simulink model "main_sys_v2_1"  (R2015a)
settings: Solver=ode23  StartTime=0.0  StopTime=Tfin  RelTol=1e-5  AbsTol=1e-5
undefined symbols (not defined in the file): init, K, param, x, x_dot, y, y_dot
settings Model: Creator=jesus  LastModifiedBy=jesus
settings SolverCC: InitialStep=1e-7  SolverResetMethod=Robust
settings DataIOCC: SaveState=on

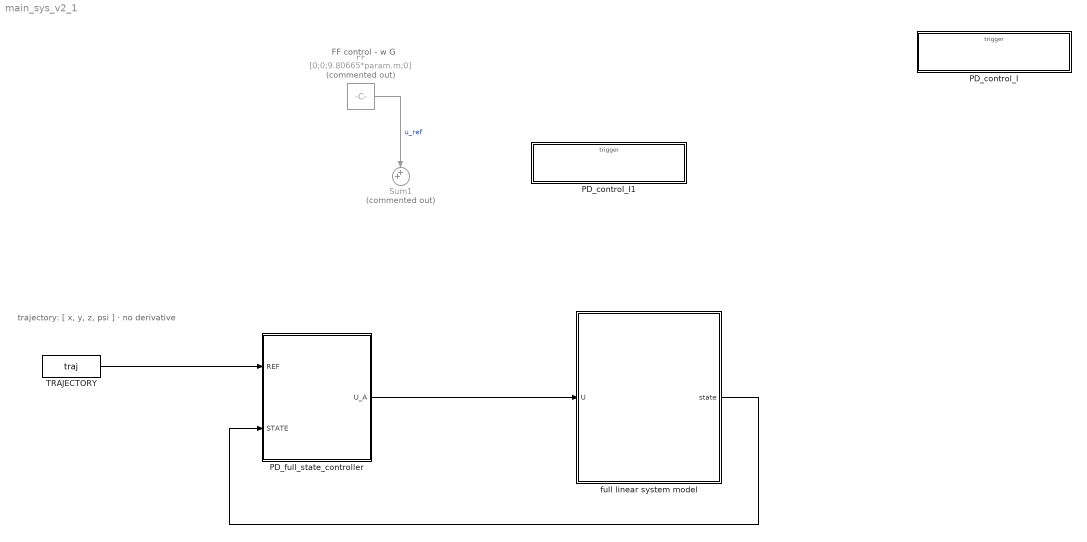
== system main_sys_v2_1 ==
  note: trajectory: [ x, y, z, psi ]
      |  · no derivative
  note: FF control - w G
  FF : Constant  Commented=on  Value=[0;0;9.80665*param.m;0]
  PD_control_I : Subsystem  TreatAsAtomicUnit=on
  PD_control_I1 : Subsystem  TreatAsAtomicUnit=on
  PD_full_state_controller : Subsystem
  Sum1 : Sum  Commented=on  Inputs=++|
  TRAJECTORY : FromWorkspace  VariableName=traj  SampleTime=param.hs  Interpolate=off  OutputAfterFinalValue=Setting to zero
  full linear system model : Subsystem
  wires:
  FF/1 -> Sum1/1  "u_ref"
  TRAJECTORY/1 -> PD_full_state_controller/1(REF)
  full linear system model/1(state) -> PD_full_state_controller/2(STATE)
  PD_full_state_controller/1(U_A) -> full linear system model/1(U)

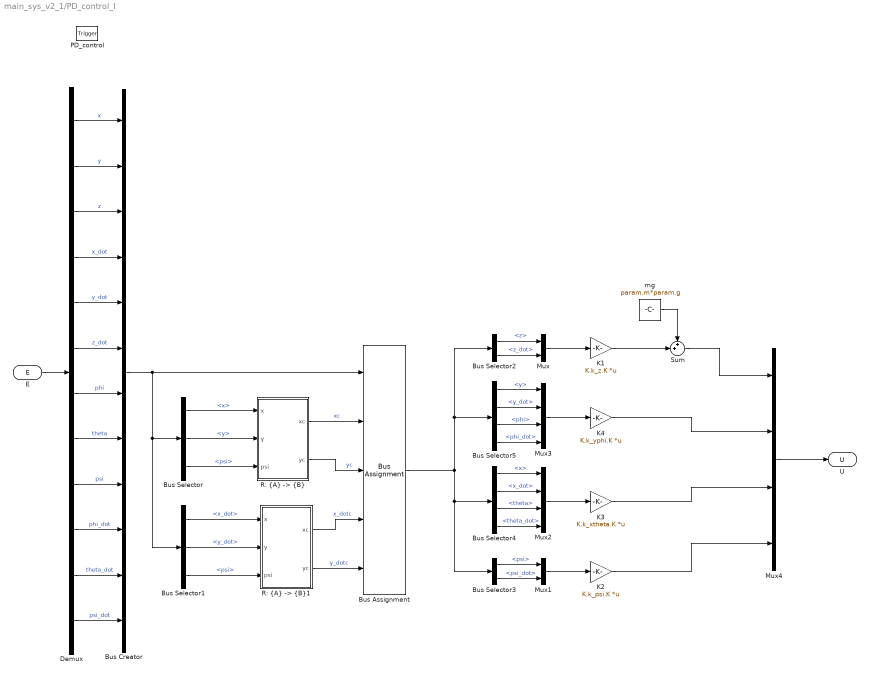
== system main_sys_v2_1/PD_control_I ==
  PD_control : TriggerPort  TriggerType=function-call  IsSimulinkFunction=on  FunctionName=PD_control
  Bus Assignment : BusAssignment  AssignedSignals=x,y,x_dot,y_dot
  Bus Creator : BusCreator  Inputs=12
  Bus Selector : BusSelector  OutputSignals=x,y,psi
  Bus Selector1 : BusSelector  OutputSignals=x_dot,y_dot,psi
  Bus Selector2 : BusSelector  OutputSignals=z,z_dot
  Bus Selector3 : BusSelector  OutputSignals=psi,psi_dot
  Bus Selector4 : BusSelector  OutputSignals=x,x_dot,theta,theta_dot
  Bus Selector5 : BusSelector  OutputSignals=y,y_dot,phi,phi_dot
  Demux : Demux  Outputs=12
  K1 : Gain  Gain=K.k_z.K  Multiplication=Matrix(K*u)
  K2 : Gain  Gain=K.k_psi.K  Multiplication=Matrix(K*u)
  K3 : Gain  Gain=K.k_xtheta.K  Multiplication=Matrix(K*u)
  K4 : Gain  Gain=K.k_yphi.K  Multiplication=Matrix(K*u)
  Mux : Mux  Inputs=2
  Mux1 : Mux  Inputs=2
  Mux2 : Mux
  Mux3 : Mux
  Mux4 : Mux
  "R: {A} -> {B}" : MATLAB Function  TreatAsAtomicUnit=on
  "R: {A} -> {B}1" : MATLAB Function  TreatAsAtomicUnit=on
  Sum : Sum  Inputs=++|
  mg : Constant  Value=param.m*param.g  SampleTime=-1
  E : ArgIn  DisableCoverage=on  PortDimensions=12  ArgumentName=E
  U : ArgOut  DisableCoverage=on  PortDimensions=4  ArgumentName=U
  wires:
  E/1 -> Demux/1
  Demux/1 -> Bus Creator/1  "x"
  Demux/2 -> Bus Creator/2  "y"
  Demux/12 -> Bus Creator/12  "psi_dot"
  Demux/7 -> Bus Creator/7  "phi"
  Demux/8 -> Bus Creator/8  "theta"
  Demux/3 -> Bus Creator/3  "z"
  Demux/4 -> Bus Creator/4  "x_dot"
  Demux/5 -> Bus Creator/5  "y_dot"
  Demux/6 -> Bus Creator/6  "z_dot"
  Demux/9 -> Bus Creator/9  "psi"
  Demux/10 -> Bus Creator/10  "phi_dot"
  Demux/11 -> Bus Creator/11  "theta_dot"
  Bus Selector/1 -> "R: {A} -> {B}"/1(x)  "<x>"
  Bus Selector/2 -> "R: {A} -> {B}"/2(y)  "<y>"
  Bus Selector/3 -> "R: {A} -> {B}"/3(psi)  "<psi>"
  "R: {A} -> {B}"/1(xc) -> Bus Assignment/2  "xc"
  "R: {A} -> {B}"/2(yc) -> Bus Assignment/3  "yc"
  Bus Creator/1 -> Bus Assignment/1, Bus Selector/1, Bus Selector1/1
  Bus Selector1/1 -> "R: {A} -> {B}1"/1(x)  "<x_dot>"
  Bus Selector1/2 -> "R: {A} -> {B}1"/2(y)  "<y_dot>"
  Bus Selector1/3 -> "R: {A} -> {B}1"/3(psi)  "<psi>"
  "R: {A} -> {B}1"/1(xc) -> Bus Assignment/4  "x_dotc"
  "R: {A} -> {B}1"/2(yc) -> Bus Assignment/5  "y_dotc"
  Bus Assignment/1 -> Bus Selector5/1, Bus Selector2/1, Bus Selector3/1, Bus Selector4/1
  Bus Selector2/1 -> Mux/1  "<z>"
  Bus Selector2/2 -> Mux/2  "<z_dot>"
  Bus Selector3/1 -> Mux1/1  "<psi>"
  Bus Selector3/2 -> Mux1/2  "<psi_dot>"
  Bus Selector5/1 -> Mux3/1  "<y>"
  Bus Selector5/2 -> Mux3/2  "<y_dot>"
  Bus Selector5/3 -> Mux3/3  "<phi>"
  Bus Selector5/4 -> Mux3/4  "<phi_dot>"
  Bus Selector4/4 -> Mux2/4  "<theta_dot>"
  Bus Selector4/3 -> Mux2/3  "<theta>"
  Bus Selector4/2 -> Mux2/2  "<x_dot>"
  Bus Selector4/1 -> Mux2/1  "<x>"
  Mux2/1 -> K3/1
  Mux1/1 -> K2/1
  Mux/1 -> K1/1
  Mux3/1 -> K4/1
  Mux4/1 -> U/1
  Sum/1 -> Mux4/1
  K1/1 -> Sum/2
  mg/1 -> Sum/1
  K4/1 -> Mux4/2
  K3/1 -> Mux4/3
  K2/1 -> Mux4/4

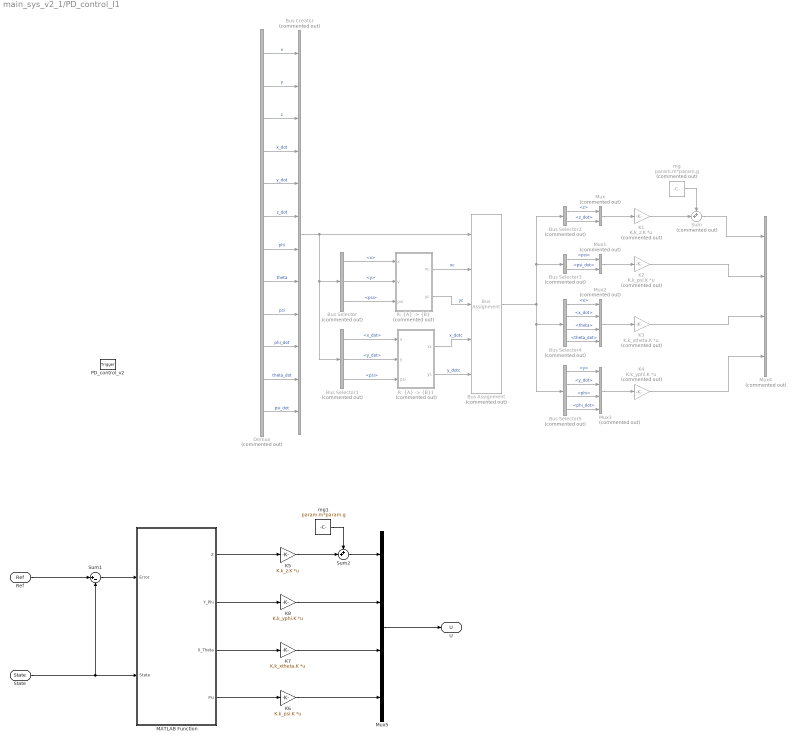
== system main_sys_v2_1/PD_control_I1 ==
  PD_control_v2 : TriggerPort  TriggerType=function-call  IsSimulinkFunction=on  FunctionName=PD_control_v2
  Bus Assignment : BusAssignment  Commented=on  AssignedSignals=x,y,x_dot,y_dot
  Bus Creator : BusCreator  Commented=on  Inputs=12
  Bus Selector : BusSelector  Commented=on  OutputSignals=x,y,psi
  Bus Selector1 : BusSelector  Commented=on  OutputSignals=x_dot,y_dot,psi
  Bus Selector2 : BusSelector  Commented=on  OutputSignals=z,z_dot
  Bus Selector3 : BusSelector  Commented=on  OutputSignals=psi,psi_dot
  Bus Selector4 : BusSelector  Commented=on  OutputSignals=x,x_dot,theta,theta_dot
  Bus Selector5 : BusSelector  Commented=on  OutputSignals=y,y_dot,phi,phi_dot
  Demux : Demux  Commented=on  Outputs=12
  K1 : Gain  Commented=on  Gain=K.k_z.K  Multiplication=Matrix(K*u)
  K2 : Gain  Commented=on  Gain=K.k_psi.K  Multiplication=Matrix(K*u)
  K3 : Gain  Commented=on  Gain=K.k_xtheta.K  Multiplication=Matrix(K*u)
  K4 : Gain  Commented=on  Gain=K.k_yphi.K  Multiplication=Matrix(K*u)
  K5 : Gain  Gain=K.k_z.K  Multiplication=Matrix(K*u)
  K6 : Gain  Gain=K.k_psi.K  Multiplication=Matrix(K*u)
  K7 : Gain  Gain=K.k_xtheta.K  Multiplication=Matrix(K*u)
  K8 : Gain  Gain=K.k_yphi.K  Multiplication=Matrix(K*u)
  MATLAB Function : MATLAB Function  TreatAsAtomicUnit=on
  Mux : Mux  Commented=on  Inputs=2
  Mux1 : Mux  Commented=on  Inputs=2
  Mux2 : Mux  Commented=on
  Mux3 : Mux  Commented=on
  Mux4 : Mux  Commented=on
  Mux5 : Mux
  "R: {A} -> {B}" : MATLAB Function  Commented=on  TreatAsAtomicUnit=on
  "R: {A} -> {B}1" : MATLAB Function  Commented=on  TreatAsAtomicUnit=on
  Sum : Sum  Commented=on  Inputs=++|
  Sum1 : Sum  Inputs=|+-
  Sum2 : Sum  Inputs=++|
  mg : Constant  Commented=on  Value=param.m*param.g  SampleTime=-1
  mg1 : Constant  Value=param.m*param.g  SampleTime=-1
  Ref : ArgIn  DisableCoverage=on  PortDimensions=12  ArgumentName=Ref
  State : ArgIn  DisableCoverage=on  Port=2  PortDimensions=12  ArgumentName=State
  U : ArgOut  DisableCoverage=on  PortDimensions=4  ArgumentName=U
  wires:
  Demux/1 -> Bus Creator/1  "x"
  Demux/2 -> Bus Creator/2  "y"
  Demux/12 -> Bus Creator/12  "psi_dot"
  Demux/7 -> Bus Creator/7  "phi"
  Demux/8 -> Bus Creator/8  "theta"
  Demux/3 -> Bus Creator/3  "z"
  Demux/4 -> Bus Creator/4  "x_dot"
  Demux/5 -> Bus Creator/5  "y_dot"
  Demux/6 -> Bus Creator/6  "z_dot"
  Demux/9 -> Bus Creator/9  "psi"
  Demux/10 -> Bus Creator/10  "phi_dot"
  Demux/11 -> Bus Creator/11  "theta_dot"
  Bus Selector/1 -> "R: {A} -> {B}"/1(x)  "<x>"
  Bus Selector/2 -> "R: {A} -> {B}"/2(y)  "<y>"
  Bus Selector/3 -> "R: {A} -> {B}"/3(psi)  "<psi>"
  "R: {A} -> {B}"/1(xc) -> Bus Assignment/2  "xc"
  "R: {A} -> {B}"/2(yc) -> Bus Assignment/3  "yc"
  Bus Creator/1 -> Bus Assignment/1, Bus Selector/1, Bus Selector1/1
  Bus Selector1/1 -> "R: {A} -> {B}1"/1(x)  "<x_dot>"
  Bus Selector1/2 -> "R: {A} -> {B}1"/2(y)  "<y_dot>"
  Bus Selector1/3 -> "R: {A} -> {B}1"/3(psi)  "<psi>"
  "R: {A} -> {B}1"/1(xc) -> Bus Assignment/4  "x_dotc"
  "R: {A} -> {B}1"/2(yc) -> Bus Assignment/5  "y_dotc"
  Bus Assignment/1 -> Bus Selector2/1, Bus Selector3/1, Bus Selector5/1, Bus Selector4/1
  Bus Selector2/1 -> Mux/1  "<z>"
  Bus Selector2/2 -> Mux/2  "<z_dot>"
  Bus Selector3/1 -> Mux1/1  "<psi>"
  Bus Selector3/2 -> Mux1/2  "<psi_dot>"
  Bus Selector5/1 -> Mux3/1  "<y>"
  Bus Selector5/2 -> Mux3/2  "<y_dot>"
  Bus Selector5/3 -> Mux3/3  "<phi>"
  Bus Selector5/4 -> Mux3/4  "<phi_dot>"
  Bus Selector4/4 -> Mux2/4  "<theta_dot>"
  Bus Selector4/3 -> Mux2/3  "<theta>"
  Bus Selector4/2 -> Mux2/2  "<x_dot>"
  Bus Selector4/1 -> Mux2/1  "<x>"
  Mux2/1 -> K3/1
  Mux1/1 -> K2/1
  Mux/1 -> K1/1
  Mux3/1 -> K4/1
  K3/1 -> Mux4/3
  K2/1 -> Mux4/2
  K4/1 -> Mux4/4
  Sum/1 -> Mux4/1
  K1/1 -> Sum/2
  mg/1 -> Sum/1
  Ref/1 -> Sum1/1
  State/1 -> Sum1/2, MATLAB Function/2(State)
  Sum1/1 -> MATLAB Function/1(Error)
  MATLAB Function/4(Psi) -> K6/1
  MATLAB Function/1(Z) -> K5/1
  MATLAB Function/3(X_Theta) -> K7/1
  MATLAB Function/2(Y_Phi) -> K8/1
  K5/1 -> Sum2/2
  mg1/1 -> Sum2/1
  K8/1 -> Mux5/2
  K7/1 -> Mux5/3
  K6/1 -> Mux5/4
  Sum2/1 -> Mux5/1
  Mux5/1 -> U/1

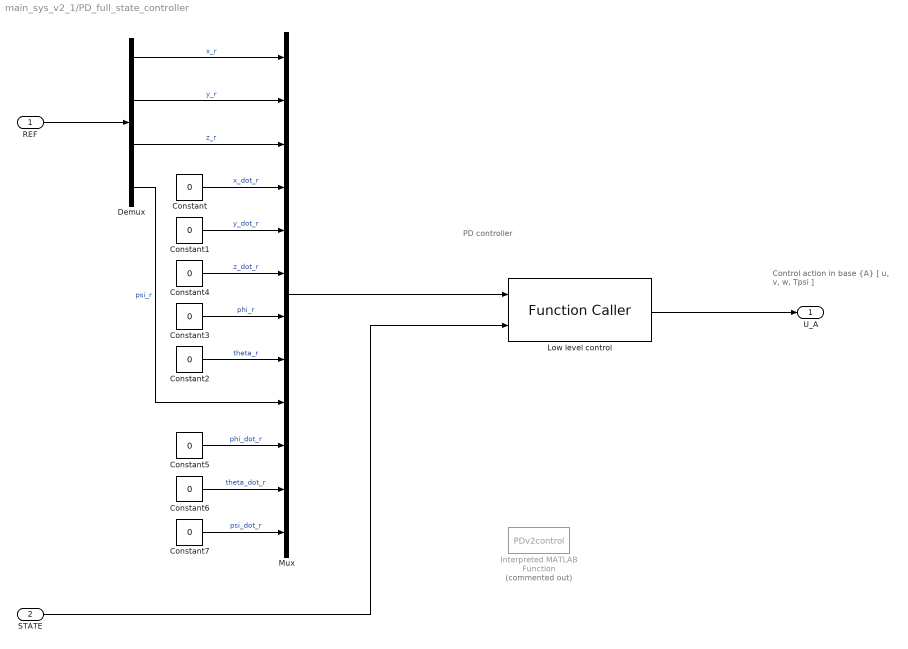
== system main_sys_v2_1/PD_full_state_controller ==
  note: Control action
      |    in base {A}
      |
      |
      |
      |
      | [ u, v, w, Tpsi ]
  note: PD controller
  REF : Inport
  STATE : Inport  Port=2
  Constant{,1..7} (8 alike) : Constant  Value=0
  Demux : Demux
  Interpreted MATLAB Function : MATLABFcn  Commented=on  MATLABFcn=PDv2control  OutputDimensions=4
  Low level control : FunctionCaller  FunctionPrototype=U = PD_control_v2(Ref,State)
  Mux : Mux  Inputs=12
  U_A : Outport
  wires:
  REF/1 -> Demux/1
  Demux/1 -> Mux/1  "x_r"
  Demux/2 -> Mux/2  "y_r"
  Demux/3 -> Mux/3  "z_r"
  STATE/1 -> Low level control/2
  Constant5/1 -> Mux/10  "phi_dot_r"
  Constant6/1 -> Mux/11  "theta_dot_r"
  Constant7/1 -> Mux/12  "psi_dot_r"
  Mux/1 -> Low level control/1
  Low level control/1 -> U_A/1
  Constant4/1 -> Mux/6  "z_dot_r"
  Constant1/1 -> Mux/5  "y_dot_r"
  Constant/1 -> Mux/4  "x_dot_r"
  Demux/4 -> Mux/9  "psi_r"
  Constant2/1 -> Mux/8  "theta_r"
  Constant3/1 -> Mux/7  "phi_r"

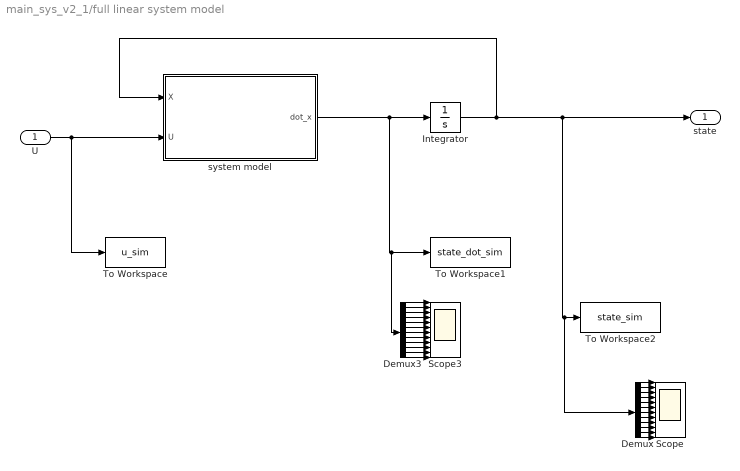
== system main_sys_v2_1/full linear system model ==
  U : Inport
  Demux : Demux  Outputs=12
  Demux3 : Demux  Outputs=12
  Integrator : Integrator  InitialCondition=init.full
  Scope : Scope  NumInputPorts=12
      settings: YMin=-5~-5~-5~-5~-5~-5~-5~-5~-5~-5~-5~-5  YMax=5~5~5~5~5~5~5~5~5~5~5~5
  Scope3 : Scope  NumInputPorts=12
      settings: YMin=-5~-5~-5~-5~-5~-5~-5~-5~-5~-5~-5~-5  YMax=5~5~5~5~5~5~5~5~5~5~5~5  SaveName=ScopeData3
  To Workspace : ToWorkspace  VariableName=u_sim  SaveFormat=Structure With Time  SampleTime=-1
  To Workspace1 : ToWorkspace  VariableName=state_dot_sim  SaveFormat=Structure With Time  SampleTime=-1
  To Workspace2 : ToWorkspace  VariableName=state_sim  SaveFormat=Structure With Time  SampleTime=-1
  system model : MATLAB Function  TreatAsAtomicUnit=on
  state : Outport
  wires:
  U/1 -> system model/2(U), To Workspace/1
  Integrator/1 -> state/1, Demux/1, To Workspace2/1, system model/1(X)
  system model/1(dot_x) -> Integrator/1, Demux3/1, To Workspace1/1
  Demux/1 -> Scope/1
  Demux/2 -> Scope/2
  Demux/3 -> Scope/3
  Demux/4 -> Scope/4
  Demux/5 -> Scope/5
  Demux/6 -> Scope/6
  Demux/7 -> Scope/7
  Demux/8 -> Scope/8
  Demux/9 -> Scope/9
  Demux/10 -> Scope/10
  Demux/11 -> Scope/11
  Demux/12 -> Scope/12
  Demux3/1 -> Scope3/1
  Demux3/2 -> Scope3/2
  Demux3/3 -> Scope3/3
  Demux3/4 -> Scope3/4
  Demux3/5 -> Scope3/5
  Demux3/6 -> Scope3/6
  Demux3/7 -> Scope3/7
  Demux3/8 -> Scope3/8
  Demux3/9 -> Scope3/9
  Demux3/10 -> Scope3/10
  Demux3/11 -> Scope3/11
  Demux3/12 -> Scope3/12

== matlab function main_sys_v2_1/PD_control_I/R: {A} -> {B} ==
  data: x input; y input; psi input; xc output; yc output
function [xc, yc] = fcn(x, y, psi)
%#codegen
% Change in cordenates from fixed frame {A} to body frame {B} of position
%  state coordenates
% · apply rotation matrix over phi (vertical) to [x] and [y]
% · the references are given in fix frame {A}, input [u] is computed in
%   body frame {B}

R = [ cos(psi) sin(psi)
     -sin(psi) cos(psi)];
a = R * [x, y]';
xc = a(1);
yc = a(2);

== matlab function main_sys_v2_1/full linear system model/system model ==
  data: X input; U input; dot_x output
function dot_x = eq_quad_lin( X, U )
% Computes the linearized dynamics model of a quadcopter

% State
    x      = X(1);     Vx   = X(4);
    y      = X(2);     Vy   = X(5);
    z      = X(3);     Vz   = X(6);

    phi    = X(7);     p    = X(10);
    theta  = X(8);     q    = X(11);
    psi    = X(9);     r    = X(12);

% Inputs
    T  = U(1);       Tphi   = U(2);
                     Ttheta = U(3);
                     Tpsi   = U(4);
                
% parameters
     m = 0.429;    g = 9.80665;   
     Ix = 0.0022375681;  Iy = 0.002985236;  Iz = 0.00480374;
    
% Equations
dot_x = zeros(12,1);

dot_x(1)  = Vx;
dot_x(2)  = Vy;
dot_x(3)  = Vz;

dot_x(4)  = -(T/m) * ( theta );
dot_x(5)  = +(T/m) * ( phi );
dot_x(6)  = -(T/m) + g;

dot_x(7)  = p;
dot_x(8)  = q;
dot_x(9)  = r;

dot_x(10) = Tphi   / Ix;
dot_x(11) = Ttheta / Iy;
dot_x(12) = Tpsi   / Iz;

end

== matlab function main_sys_v2_1/PD_control_I/R: {A} -> {B}1 ==
  data: x input; y input; psi input; xc output; yc output
function [xc, yc] = fcn(x, y, psi)
%#codegen
% Change in cordenates from fixed frame {A} to body frame {B} of position
%  state coordenates
% · apply rotation matrix over phi (vertical) to [x] and [y]
% · the references are given in fix frame {A}, input [u] is computed in
%   body frame {B}

R = [ cos(psi) sin(psi)
     -sin(psi) cos(psi)];
a = R * [x; y];
xc = a(1); 
yc = a(2);

== matlab function main_sys_v2_1/PD_control_I1/R: {A} -> {B} ==
  data: x input; y input; psi input; xc output; yc output
function [xc, yc] = fcn(x, y, psi)
%#codegen
% Change in cordenates from fixed frame {A} to body frame {B} of position
%  state coordenates
% · apply rotation matrix over phi (vertical) to [x] and [y]
% · the references are given in fix frame {A}, input [u] is computed in
%   body frame {B}

R = [ cos(psi) sin(psi)
     -sin(psi) cos(psi)];
a = R * [x, y]';
xc = a(1);
yc = a(2);

== matlab function main_sys_v2_1/PD_control_I1/R: {A} -> {B}1 ==
  data: x input; y input; psi input; xc output; yc output
function [xc, yc] = fcn(x, y, psi)
%#codegen
% Change in cordenates from fixed frame {A} to body frame {B} of position
%  state coordenates
% · apply rotation matrix over phi (vertical) to [x] and [y]
% · the references are given in fix frame {A}, input [u] is computed in
%   body frame {B}

R = [ cos(psi) sin(psi)
     -sin(psi) cos(psi)];
a = R * [x; y];
xc = a(1); 
yc = a(2);

== matlab function main_sys_v2_1/PD_control_I1/MATLAB Function ==
  data: Error input; State input; Z output; Y_Phi output; X_Theta output; Psi output
function [Z, Y_Phi, X_Theta, Psi] = fcn(Error, State)
%#codegen

% Inputs
    % Error = Ref - State
    x_e = Error(1);       x_dot_e = Error(4);
    y_e = Error(2);       y_dot_e = Error(5);
    z_e = Error(3);       z_dot_e = Error(6);

    phi_e   = Error(7);   phi_dot_e   = Error(10);
    theta_e = Error(8);   theta_dot_e = Error(11);
    psi_e   = Error(9);   psi_dot_e   = Error(12);
    
    % State
    x = State(1);       x_dot = State(4);
    y = State(2);       y_dot = State(5);
    z = State(3);       z_dot = State(6);

    phi   = State(7);   phi_dot   = State(10);
    theta = State(8);   theta_dot = State(11);
    psi   = State(9);   psi_dot   = State(12);
    
% Change of base
    % rotation matrix
    R = [ c(theta)*c(psi), s(phi)*s(theta)*c(psi)-c(phi)*s(psi), c(phi)*s(theta)*c(psi)+s(phi)*s(psi);
          c(theta)*s(psi), s(phi)*s(theta)*s(psi)+c(phi)*c(psi), c(phi)*s(theta)*s(psi)-s(phi)*c(psi);
          -s(theta),       s(phi)*c(theta),                      c(phi)*c(theta)                      ];
    
    xyz_e_B = R * [x_e; y_e; z_e];
    xyz_dot_e_B = R * [x_dot_e; y_dot_e; z_dot_e];

% Output - vector subsystems
    % 'x-theta'
    X_Theta = [xyz_e_B(1); xyz_dot_e_B(1); theta_e; theta_dot_e];
    % 'y-phi'
    Y_Phi = [xyz_e_B(2); xyz_dot_e_B(2); phi_e; phi_dot_e];
    % 'z'
    %Z = [xyz_e_B(3); xyz_dot_e_B(3)];
    Z = [z_e; z_dot_e];
    % 'psi'
    Psi = [psi_e; psi_dot_e];
end

function y = s(angle)
    y = sin(angle);
end

function y = c(angle)
    y = cos(angle);
end
